simulink model "basis3"  (Simulink 6.6)
settings: Solver=ode45  StartTime=0.0  StopTime=inf  RelTol=1e-3
libraries: simulink x57, dspstat3 x3
settings Model: Creator=Paul.Dourbal  LastModifiedBy=Paul.Dourbal

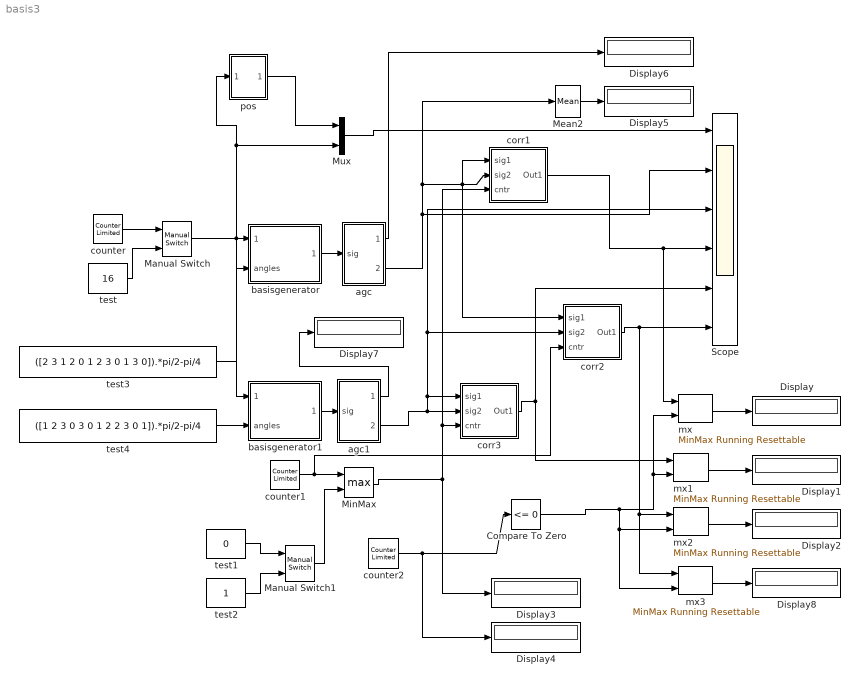
== system basis3 ==
  Compare To Zero : simulink/Logic and Bit Operations/Compare To Zero  SystemSampleTime=-1  relop=<=  LogicOutDataTypeMode=uint8  ZeroCross=off
  Display{,1..8} (9 alike) : Display
  Manual Switch : simulink/Signal Routing/Manual Switch  SystemSampleTime=-1  sw=1  action=0  varsize=off
  Manual Switch1 : simulink/Signal Routing/Manual Switch  SystemSampleTime=-1  sw=0  action=0  varsize=off
  Mean2 : dspstat3/Mean  DialogController=dspDDGCreate  DialogControllerArgs=DataTag0  run=on  reset_popup=None  roundingMode=Floor  overflowMode=on
  MinMax : MinMax  Function=max  Inputs=2  SampleTime=1
  Mux : Mux  Inputs=2
  Scope : Scope  NumInputPorts=6
      settings: TimeRange=102200  YMin=0~-1.25~-1.25~-0.1~-1~-1  YMax=70~1.25~1~1~1~2
  agc : Subsystem
  agc1 : Subsystem
  basisgenerator : Subsystem
  basisgenerator1 : Subsystem
  corr1 : Subsystem
  corr2 : Subsystem
  corr3 : Subsystem
  counter : simulink/Sources/Counter Limited  SystemSampleTime=-1  uplimit=2^(3+3)-1  tsamp=1
  counter1 : simulink/Sources/Counter Limited  SystemSampleTime=-1  uplimit=2^(3+3)-1  tsamp=256
  counter2 : simulink/Sources/Counter Limited  SystemSampleTime=-1  uplimit=2^(3+3)-1  tsamp=1024
  mx : simulink/Math Operations/MinMax Running Resettable  SystemSampleTime=-1  Function=max  vinit=0.0
  mx1 : simulink/Math Operations/MinMax Running Resettable  SystemSampleTime=-1  Function=max  vinit=0.0
  mx2 : simulink/Math Operations/MinMax Running Resettable  SystemSampleTime=-1  Function=max  vinit=0.0
  mx3 : simulink/Math Operations/MinMax Running Resettable  SystemSampleTime=-1  Function=min  vinit=0.0
  pos : Subsystem
  test : Constant  Value=16  OutDataTypeMode=uint8
  test1 : Constant  Value=0  OutDataTypeMode=uint8
  test2 : Constant  OutDataTypeMode=uint8
  test3 : Constant  Value=([2 3 1 2 0 1 2 3 0 1 3 0]).*pi/2-pi/4  OutDataTypeMode=double
  test4 : Constant  Value=([1 2 3 0 3 0 1 2 2 3 0 1]).*pi/2-pi/4  OutDataTypeMode=double
  wires:
  test/1 -> Manual Switch/2
  counter/1 -> Manual Switch/1
  Manual Switch/1 -> basisgenerator/1(counter), basisgenerator1/1(counter), pos/1(In1), Mux/2
  pos/1(Out1) -> Mux/1
  Mux/1 -> Scope/1
  corr1/1(Out1) -> Scope/4, mx/1
  corr3/1(Out1) -> Scope/5, mx1/1
  corr2/1(Out1) -> Scope/6, mx2/1, mx3/1
  counter1/1 -> MinMax/1, corr2/3(cntr)
  mx/1 -> Display/1
  mx1/1 -> Display1/1
  mx2/1 -> Display2/1
  Compare To Zero/1 -> mx/2, mx1/2, mx2/2, mx3/2
  counter2/1 -> Compare To Zero/1, Display4/1
  agc/2(out) -> Scope/2, corr1/2(sig2), corr1/1(sig1), corr2/1(sig1), Mean2/1
  agc1/2(out) -> Scope/3, corr2/2(sig2), corr3/1(sig1), corr3/2(sig2)
  Mean2/1 -> Display5/1
  agc/1(mean) -> Display6/1
  basisgenerator/1(samples) -> agc/1(sig)
  basisgenerator1/1(samples) -> agc1/1(sig)
  agc1/1(mean) -> Display7/1
  MinMax/1 -> corr1/3(cntr), corr3/3(cntr), Display3/1
  Manual Switch1/1 -> MinMax/2
  test1/1 -> Manual Switch1/1
  test2/1 -> Manual Switch1/2
  test4/1 -> basisgenerator1/2(angles)
  test3/1 -> basisgenerator/2(angles)
  mx3/1 -> Display8/1

== system basis3/agc ==
  sig : Inport
  Mean : dspstat3/Mean  DialogController=dspDDGCreate  DialogControllerArgs=DataTag1  run=on  reset_popup=None  roundingMode=Nearest  overflowMode=on
  Subtract : Sum  Inputs=+-  OutScaling=2^-10  SampleTime=1
  mean : Outport
  out : Outport  Port=2
  wires:
  sig/1 -> Subtract/1, Mean/1
  Mean/1 -> Subtract/2, mean/1
  Subtract/1 -> out/1

== system basis3/agc1 ==
  sig : Inport
  Mean : dspstat3/Mean  DialogController=dspDDGCreate  DialogControllerArgs=DataTag2  run=on  reset_popup=None  roundingMode=Nearest  overflowMode=on
  Subtract : Sum  Inputs=+-  OutScaling=2^-10  SampleTime=1
  mean : Outport
  out : Outport  Port=2
  wires:
  sig/1 -> Subtract/1, Mean/1
  Mean/1 -> Subtract/2, mean/1
  Subtract/1 -> out/1

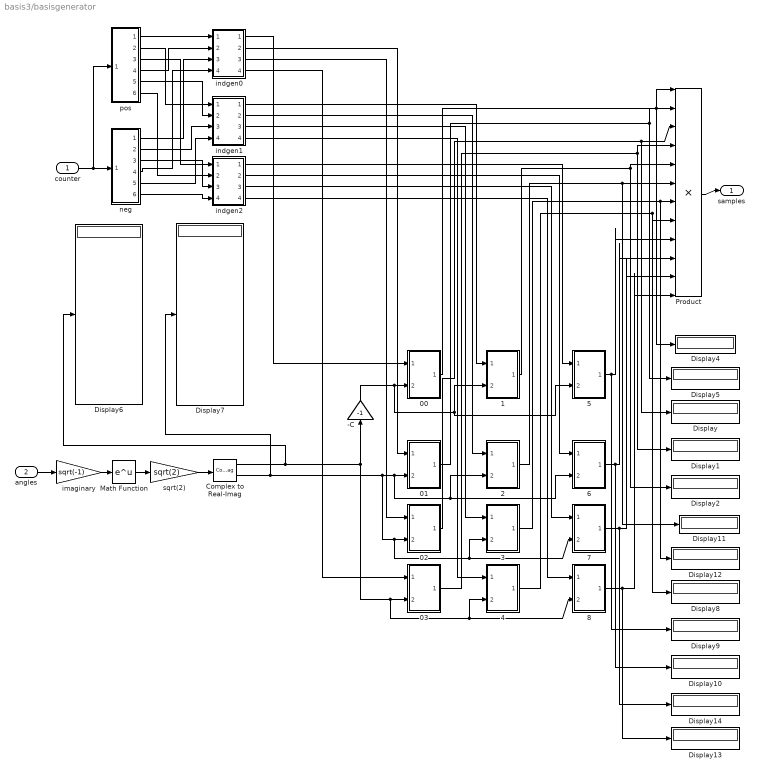
== system basis3/basisgenerator ==
  counter : Inport
  angles : Inport  Port=2
  -C : Gain  Orientation=up  Gain=-1
  00 : Subsystem
  01 : Subsystem
  02 : Subsystem
  03 : Subsystem
  1 : Subsystem
  2 : Subsystem
  3 : Subsystem
  4 : Subsystem
  5 : Subsystem
  6 : Subsystem
  7 : Subsystem
  8 : Subsystem
  Complex to Real-Imag : ComplexToRealImag
  Display{,1..2,4..14} (14 alike) : Display
  Math Function : Math  OutputSignalType=complex  SaturateOnIntegerOverflow=on
  Product : Product  Inputs=12  RndMeth=Zero
  imaginary : Gain  Gain=sqrt(-1)
  indgen0 : Subsystem
  indgen1 : Subsystem
  indgen2 : Subsystem
  neg : Subsystem
  pos : Subsystem
  sqrt(2) : Gain  Gain=sqrt(2)
  samples : Outport
  wires:
  8/1(Out1) -> Product/12, Display13/1
  7/1(Out1) -> Product/11, Display14/1
  6/1(Out1) -> Product/10, Display10/1
  5/1(Out1) -> Product/9, Display9/1
  4/1(Out1) -> Product/8, Display8/1
  3/1(Out1) -> Product/7, Display12/1
  2/1(Out1) -> Product/6, Display11/1
  1/1(Out1) -> Product/5, Display2/1
  03/1(Out1) -> Product/4, Display1/1
  02/1(Out1) -> Product/3, Display/1
  01/1(Out1) -> Product/2, Display5/1
  00/1(Out1) -> Product/1, Display4/1
  indgen2/4(Out4) -> 8/1(In1)
  indgen2/3(Out3) -> 7/1(In1)
  indgen2/2(Out2) -> 6/1(In1)
  indgen2/1(Out1) -> 5/1(In1)
  indgen1/4(Out4) -> 4/1(In1)
  indgen1/3(Out3) -> 3/1(In1)
  indgen1/2(Out2) -> 2/1(In1)
  indgen1/1(Out1) -> 1/1(In1)
  indgen0/4(Out4) -> 03/1(In1)
  indgen0/3(Out3) -> 02/1(In1)
  indgen0/2(Out2) -> 01/1(In1)
  indgen0/1(Out1) -> 00/1(In1)
  -C/1 -> 00/2(In2), 1/2(In2), 5/2(In2)
  neg/6(Out6) -> indgen2/4(In4)
  neg/3(Out3) -> indgen2/3(In3)
  pos/6(Out6) -> indgen2/2(In2)
  pos/3(Out3) -> indgen2/1(In1)
  neg/5(Out5) -> indgen1/4(In4)
  neg/2(Out2) -> indgen1/3(In3)
  pos/5(Out5) -> indgen1/2(In2)
  pos/2(Out2) -> indgen1/1(In1)
  neg/4(Out4) -> indgen0/4(In4)
  neg/1(Out1) -> indgen0/3(In3)
  pos/4(Out4) -> indgen0/2(In2)
  pos/1(Out1) -> indgen0/1(In1)
  Complex to Real-Imag/2 -> 01/2(In2), 2/2(In2), 6/2(In2), 02/2(In2), 3/2(In2), 7/2(In2), Display7/1
  Complex to Real-Imag/1 -> -C/1, 03/2(In2), 4/2(In2), 8/2(In2), Display6/1
  sqrt(2)/1 -> Complex to Real-Imag/1
  Math Function/1 -> sqrt(2)/1
  imaginary/1 -> Math Function/1
  counter/1 -> neg/1(In1), pos/1(In1)
  Product/1 -> samples/1
  angles/1 -> imaginary/1

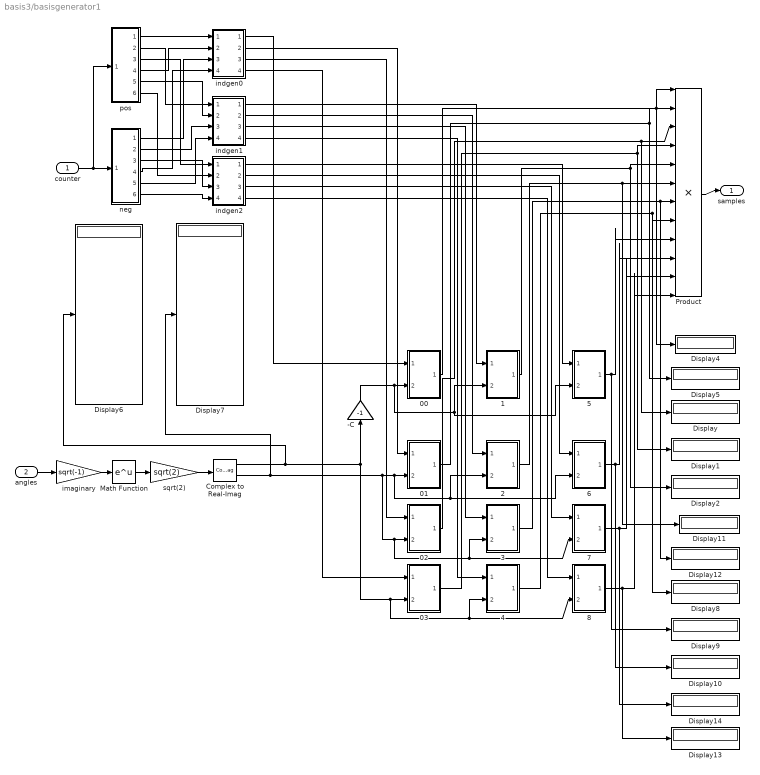
== system basis3/basisgenerator1 ==
  counter : Inport
  angles : Inport  Port=2
  -C : Gain  Orientation=up  Gain=-1
  00 : Subsystem
  01 : Subsystem
  02 : Subsystem
  03 : Subsystem
  1 : Subsystem
  2 : Subsystem
  3 : Subsystem
  4 : Subsystem
  5 : Subsystem
  6 : Subsystem
  7 : Subsystem
  8 : Subsystem
  Complex to Real-Imag : ComplexToRealImag
  Display{,1..2,4..14} (14 alike) : Display
  Math Function : Math  OutputSignalType=complex  SaturateOnIntegerOverflow=on
  Product : Product  Inputs=12  RndMeth=Zero
  imaginary : Gain  Gain=sqrt(-1)
  indgen0 : Subsystem
  indgen1 : Subsystem
  indgen2 : Subsystem
  neg : Subsystem
  pos : Subsystem
  sqrt(2) : Gain  Gain=sqrt(2)
  samples : Outport
  wires:
  8/1(Out1) -> Product/12, Display13/1
  7/1(Out1) -> Product/11, Display14/1
  6/1(Out1) -> Product/10, Display10/1
  5/1(Out1) -> Product/9, Display9/1
  4/1(Out1) -> Product/8, Display8/1
  3/1(Out1) -> Product/7, Display12/1
  2/1(Out1) -> Product/6, Display11/1
  1/1(Out1) -> Product/5, Display2/1
  03/1(Out1) -> Product/4, Display1/1
  02/1(Out1) -> Product/3, Display/1
  01/1(Out1) -> Product/2, Display5/1
  00/1(Out1) -> Product/1, Display4/1
  indgen2/4(Out4) -> 8/1(In1)
  indgen2/3(Out3) -> 7/1(In1)
  indgen2/2(Out2) -> 6/1(In1)
  indgen2/1(Out1) -> 5/1(In1)
  indgen1/4(Out4) -> 4/1(In1)
  indgen1/3(Out3) -> 3/1(In1)
  indgen1/2(Out2) -> 2/1(In1)
  indgen1/1(Out1) -> 1/1(In1)
  indgen0/4(Out4) -> 03/1(In1)
  indgen0/3(Out3) -> 02/1(In1)
  indgen0/2(Out2) -> 01/1(In1)
  indgen0/1(Out1) -> 00/1(In1)
  -C/1 -> 00/2(In2), 1/2(In2), 5/2(In2)
  neg/6(Out6) -> indgen2/4(In4)
  neg/3(Out3) -> indgen2/3(In3)
  pos/6(Out6) -> indgen2/2(In2)
  pos/3(Out3) -> indgen2/1(In1)
  neg/5(Out5) -> indgen1/4(In4)
  neg/2(Out2) -> indgen1/3(In3)
  pos/5(Out5) -> indgen1/2(In2)
  pos/2(Out2) -> indgen1/1(In1)
  neg/4(Out4) -> indgen0/4(In4)
  neg/1(Out1) -> indgen0/3(In3)
  pos/4(Out4) -> indgen0/2(In2)
  pos/1(Out1) -> indgen0/1(In1)
  Complex to Real-Imag/2 -> 01/2(In2), 2/2(In2), 6/2(In2), 02/2(In2), 3/2(In2), 7/2(In2), Display7/1
  Complex to Real-Imag/1 -> -C/1, 03/2(In2), 4/2(In2), 8/2(In2), Display6/1
  sqrt(2)/1 -> Complex to Real-Imag/1
  Math Function/1 -> sqrt(2)/1
  imaginary/1 -> Math Function/1
  counter/1 -> neg/1(In1), pos/1(In1)
  Product/1 -> samples/1
  angles/1 -> imaginary/1

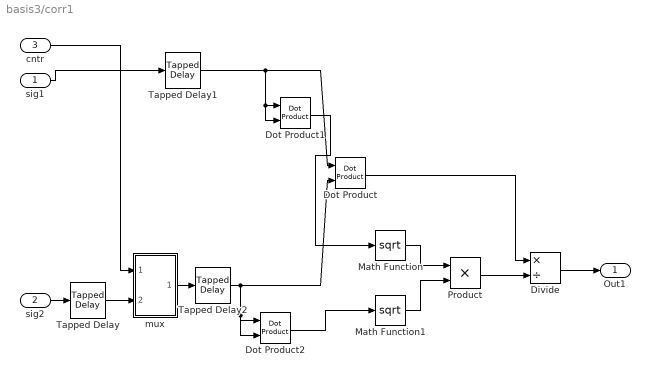
== system basis3/corr1 ==
  sig1 : Inport
  sig2 : Inport  Port=2
  cntr : Inport  Port=3
  Divide : Product  Inputs=*/  OutScaling=2^-10
  Dot Product : simulink/Math Operations/Dot Product  InputSameDT=on  OutDataType=sfix(16)  OutScaling=2^-10  DoSatur=off
  Dot Product1 : simulink/Math Operations/Dot Product  InputSameDT=on  OutDataType=sfix(16)  OutScaling=2^-10  DoSatur=off
  Dot Product2 : simulink/Math Operations/Dot Product  InputSameDT=on  OutDataType=sfix(16)  OutScaling=2^-10  DoSatur=off
  Math Function : Math  Operator=sqrt  SaturateOnIntegerOverflow=on
  Math Function1 : Math  Operator=sqrt  SaturateOnIntegerOverflow=on
  Product : Product  RndMeth=Zero
  Tapped Delay : simulink/Discrete/Tapped Delay  vinit=0.0  samptime=1  NumDelays=64  DelayOrder=Oldest  includeCurrent=off
  Tapped Delay1 : simulink/Discrete/Tapped Delay  vinit=0.0  samptime=1  NumDelays=64  DelayOrder=Oldest  includeCurrent=off
  Tapped Delay2 : simulink/Discrete/Tapped Delay  vinit=0.0  samptime=1  NumDelays=64  DelayOrder=Oldest  includeCurrent=off
  mux : Subsystem
  Out1 : Outport
  wires:
  Divide/1 -> Out1/1
  sig1/1 -> Tapped Delay1/1
  sig2/1 -> Tapped Delay/1
  Tapped Delay/1 -> mux/2(In2)
  cntr/1 -> mux/1(In1)
  mux/1(Out1) -> Tapped Delay2/1
  Tapped Delay1/1 -> Dot Product/1, Dot Product1/1, Dot Product1/2
  Tapped Delay2/1 -> Dot Product/2, Dot Product2/2, Dot Product2/1
  Math Function/1 -> Product/1
  Math Function1/1 -> Product/2
  Product/1 -> Divide/2
  Dot Product1/1 -> Math Function/1
  Dot Product2/1 -> Math Function1/1
  Dot Product/1 -> Divide/1

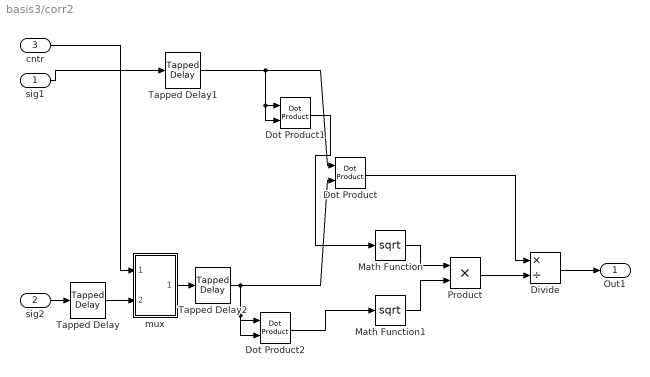
== system basis3/corr2 ==
  sig1 : Inport
  sig2 : Inport  Port=2
  cntr : Inport  Port=3
  Divide : Product  Inputs=*/  OutScaling=2^-10
  Dot Product : simulink/Math Operations/Dot Product  InputSameDT=on  OutDataType=sfix(16)  OutScaling=2^-10  DoSatur=off
  Dot Product1 : simulink/Math Operations/Dot Product  InputSameDT=on  OutDataType=sfix(16)  OutScaling=2^-10  DoSatur=off
  Dot Product2 : simulink/Math Operations/Dot Product  InputSameDT=on  OutDataType=sfix(16)  OutScaling=2^-10  DoSatur=off
  Math Function : Math  Operator=sqrt  SaturateOnIntegerOverflow=on
  Math Function1 : Math  Operator=sqrt  SaturateOnIntegerOverflow=on
  Product : Product  RndMeth=Zero
  Tapped Delay : simulink/Discrete/Tapped Delay  vinit=0.0  samptime=1  NumDelays=64  DelayOrder=Oldest  includeCurrent=off
  Tapped Delay1 : simulink/Discrete/Tapped Delay  vinit=0.0  samptime=1  NumDelays=64  DelayOrder=Oldest  includeCurrent=off
  Tapped Delay2 : simulink/Discrete/Tapped Delay  vinit=0.0  samptime=1  NumDelays=64  DelayOrder=Oldest  includeCurrent=off
  mux : Subsystem
  Out1 : Outport
  wires:
  Divide/1 -> Out1/1
  sig1/1 -> Tapped Delay1/1
  sig2/1 -> Tapped Delay/1
  Tapped Delay/1 -> mux/2(In2)
  cntr/1 -> mux/1(In1)
  mux/1(Out1) -> Tapped Delay2/1
  Tapped Delay1/1 -> Dot Product/1, Dot Product1/1, Dot Product1/2
  Tapped Delay2/1 -> Dot Product/2, Dot Product2/2, Dot Product2/1
  Math Function/1 -> Product/1
  Math Function1/1 -> Product/2
  Product/1 -> Divide/2
  Dot Product1/1 -> Math Function/1
  Dot Product2/1 -> Math Function1/1
  Dot Product/1 -> Divide/1

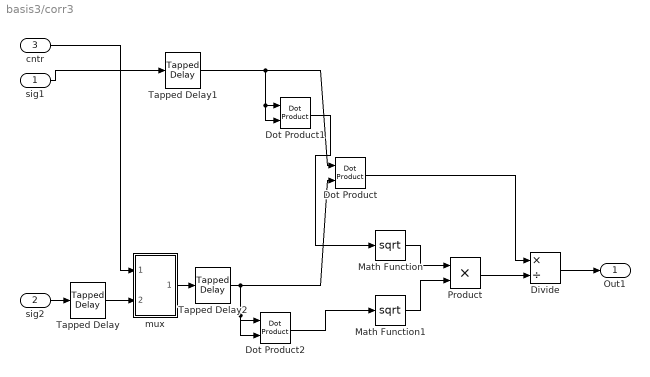
== system basis3/corr3 ==
  sig1 : Inport
  sig2 : Inport  Port=2
  cntr : Inport  Port=3
  Divide : Product  Inputs=*/  OutScaling=2^-10
  Dot Product : simulink/Math Operations/Dot Product  InputSameDT=on  OutDataType=sfix(16)  OutScaling=2^-10  DoSatur=off
  Dot Product1 : simulink/Math Operations/Dot Product  InputSameDT=on  OutDataType=sfix(16)  OutScaling=2^-10  DoSatur=off
  Dot Product2 : simulink/Math Operations/Dot Product  InputSameDT=on  OutDataType=sfix(16)  OutScaling=2^-10  DoSatur=off
  Math Function : Math  Operator=sqrt  SaturateOnIntegerOverflow=on
  Math Function1 : Math  Operator=sqrt  SaturateOnIntegerOverflow=on
  Product : Product  RndMeth=Zero
  Tapped Delay : simulink/Discrete/Tapped Delay  vinit=0.0  samptime=1  NumDelays=64  DelayOrder=Oldest  includeCurrent=off
  Tapped Delay1 : simulink/Discrete/Tapped Delay  vinit=0.0  samptime=1  NumDelays=64  DelayOrder=Oldest  includeCurrent=off
  Tapped Delay2 : simulink/Discrete/Tapped Delay  vinit=0.0  samptime=1  NumDelays=64  DelayOrder=Oldest  includeCurrent=off
  mux : Subsystem
  Out1 : Outport
  wires:
  Divide/1 -> Out1/1
  sig1/1 -> Tapped Delay1/1
  sig2/1 -> Tapped Delay/1
  Tapped Delay/1 -> mux/2(In2)
  cntr/1 -> mux/1(In1)
  mux/1(Out1) -> Tapped Delay2/1
  Tapped Delay1/1 -> Dot Product/1, Dot Product1/1, Dot Product1/2
  Tapped Delay2/1 -> Dot Product/2, Dot Product2/2, Dot Product2/1
  Math Function/1 -> Product/1
  Math Function1/1 -> Product/2
  Product/1 -> Divide/2
  Dot Product1/1 -> Math Function/1
  Dot Product2/1 -> Math Function1/1
  Dot Product/1 -> Divide/1

== system basis3/pos ==
  In1 : Inport  Orientation=up
  Extract Bits3 : simulink/Logic and Bit Operations/Extract Bits  SystemSampleTime=-1  bitsToExtract=Range of bits  numBits=8  bitIdxRange=[2 2]  outScalingMode=Treat bit field as an integer
  Extract Bits4 : simulink/Logic and Bit Operations/Extract Bits  SystemSampleTime=-1  bitsToExtract=Range of bits  numBits=8  bitIdxRange=[1 1]  outScalingMode=Treat bit field as an integer
  Extract Bits5 : simulink/Logic and Bit Operations/Extract Bits  SystemSampleTime=-1  bitsToExtract=Range of bits  numBits=8  bitIdxRange=[0 0]  outScalingMode=Treat bit field as an integer
  ws : Subsystem
  Out1 : Outport
  wires:
  Extract Bits5/1 -> ws/1(in0)
  In1/1 -> Extract Bits3/1, Extract Bits5/1, Extract Bits4/1
  Extract Bits4/1 -> ws/2(in1)
  Extract Bits3/1 -> ws/3(in2)
  ws/1(Out1) -> Out1/1

== system basis3/basisgenerator/00 ==
  In1 : Inport
  In2 : Inport  Port=2
  C : MultiPortSwitch  Inputs=12  zeroidx=on
  Demux3 : Demux  Outputs=12
  Out1 : Outport
  wires:
  Demux3/1 -> C/2
  Demux3/2 -> C/3
  Demux3/3 -> C/4
  Demux3/4 -> C/5
  Demux3/5 -> C/6
  Demux3/6 -> C/7
  Demux3/7 -> C/8
  Demux3/8 -> C/9
  Demux3/9 -> C/10
  Demux3/10 -> C/11
  Demux3/11 -> C/12
  Demux3/12 -> C/13
  In1/1 -> C/1
  C/1 -> Out1/1
  In2/1 -> Demux3/1

== system basis3/basisgenerator/01 ==
  In1 : Inport
  In2 : Inport  Port=2
  C : MultiPortSwitch  Inputs=12  zeroidx=on
  Demux3 : Demux  Outputs=12
  Out1 : Outport
  wires:
  Demux3/1 -> C/2
  Demux3/2 -> C/3
  Demux3/3 -> C/4
  Demux3/4 -> C/5
  Demux3/5 -> C/6
  Demux3/6 -> C/7
  Demux3/7 -> C/8
  Demux3/8 -> C/9
  Demux3/9 -> C/10
  Demux3/10 -> C/11
  Demux3/11 -> C/12
  Demux3/12 -> C/13
  In1/1 -> C/1
  C/1 -> Out1/1
  In2/1 -> Demux3/1

== system basis3/basisgenerator/02 ==
  In1 : Inport
  In2 : Inport  Port=2
  C : MultiPortSwitch  Inputs=12  zeroidx=on
  Demux3 : Demux  Outputs=12
  Out1 : Outport
  wires:
  Demux3/1 -> C/2
  Demux3/2 -> C/3
  Demux3/3 -> C/4
  Demux3/4 -> C/5
  Demux3/5 -> C/6
  Demux3/6 -> C/7
  Demux3/7 -> C/8
  Demux3/8 -> C/9
  Demux3/9 -> C/10
  Demux3/10 -> C/11
  Demux3/11 -> C/12
  Demux3/12 -> C/13
  In1/1 -> C/1
  C/1 -> Out1/1
  In2/1 -> Demux3/1

== system basis3/basisgenerator/03 ==
  In1 : Inport
  In2 : Inport  Port=2
  C : MultiPortSwitch  Inputs=12  zeroidx=on
  Demux3 : Demux  Outputs=12
  Out1 : Outport
  wires:
  Demux3/1 -> C/2
  Demux3/2 -> C/3
  Demux3/3 -> C/4
  Demux3/4 -> C/5
  Demux3/5 -> C/6
  Demux3/6 -> C/7
  Demux3/7 -> C/8
  Demux3/8 -> C/9
  Demux3/9 -> C/10
  Demux3/10 -> C/11
  Demux3/11 -> C/12
  Demux3/12 -> C/13
  In1/1 -> C/1
  C/1 -> Out1/1
  In2/1 -> Demux3/1

== system basis3/basisgenerator/1 ==
  In1 : Inport
  In2 : Inport  Port=2
  C : MultiPortSwitch  Inputs=12  zeroidx=on
  Demux3 : Demux  Outputs=12
  Out1 : Outport
  wires:
  Demux3/1 -> C/2
  Demux3/2 -> C/3
  Demux3/3 -> C/4
  Demux3/4 -> C/5
  Demux3/5 -> C/6
  Demux3/6 -> C/7
  Demux3/7 -> C/8
  Demux3/8 -> C/9
  Demux3/9 -> C/10
  Demux3/10 -> C/11
  Demux3/11 -> C/12
  Demux3/12 -> C/13
  In1/1 -> C/1
  C/1 -> Out1/1
  In2/1 -> Demux3/1

== system basis3/basisgenerator/2 ==
  In1 : Inport
  In2 : Inport  Port=2
  C : MultiPortSwitch  Inputs=12  zeroidx=on
  Demux3 : Demux  Outputs=12
  Out1 : Outport
  wires:
  Demux3/1 -> C/2
  Demux3/2 -> C/3
  Demux3/3 -> C/4
  Demux3/4 -> C/5
  Demux3/5 -> C/6
  Demux3/6 -> C/7
  Demux3/7 -> C/8
  Demux3/8 -> C/9
  Demux3/9 -> C/10
  Demux3/10 -> C/11
  Demux3/11 -> C/12
  Demux3/12 -> C/13
  In1/1 -> C/1
  C/1 -> Out1/1
  In2/1 -> Demux3/1

== system basis3/basisgenerator/3 ==
  In1 : Inport
  In2 : Inport  Port=2
  C : MultiPortSwitch  Inputs=12  zeroidx=on
  Demux3 : Demux  Outputs=12
  Out1 : Outport
  wires:
  Demux3/1 -> C/2
  Demux3/2 -> C/3
  Demux3/3 -> C/4
  Demux3/4 -> C/5
  Demux3/5 -> C/6
  Demux3/6 -> C/7
  Demux3/7 -> C/8
  Demux3/8 -> C/9
  Demux3/9 -> C/10
  Demux3/10 -> C/11
  Demux3/11 -> C/12
  Demux3/12 -> C/13
  In1/1 -> C/1
  C/1 -> Out1/1
  In2/1 -> Demux3/1

== system basis3/basisgenerator/4 ==
  In1 : Inport
  In2 : Inport  Port=2
  C : MultiPortSwitch  Inputs=12  zeroidx=on
  Demux3 : Demux  Outputs=12
  Out1 : Outport
  wires:
  Demux3/1 -> C/2
  Demux3/2 -> C/3
  Demux3/3 -> C/4
  Demux3/4 -> C/5
  Demux3/5 -> C/6
  Demux3/6 -> C/7
  Demux3/7 -> C/8
  Demux3/8 -> C/9
  Demux3/9 -> C/10
  Demux3/10 -> C/11
  Demux3/11 -> C/12
  Demux3/12 -> C/13
  In1/1 -> C/1
  C/1 -> Out1/1
  In2/1 -> Demux3/1

== system basis3/basisgenerator/5 ==
  In1 : Inport
  In2 : Inport  Port=2
  C : MultiPortSwitch  Inputs=12  zeroidx=on
  Demux3 : Demux  Outputs=12
  Out1 : Outport
  wires:
  Demux3/1 -> C/2
  Demux3/2 -> C/3
  Demux3/3 -> C/4
  Demux3/4 -> C/5
  Demux3/5 -> C/6
  Demux3/6 -> C/7
  Demux3/7 -> C/8
  Demux3/8 -> C/9
  Demux3/9 -> C/10
  Demux3/10 -> C/11
  Demux3/11 -> C/12
  Demux3/12 -> C/13
  In1/1 -> C/1
  C/1 -> Out1/1
  In2/1 -> Demux3/1

== system basis3/basisgenerator/6 ==
  In1 : Inport
  In2 : Inport  Port=2
  C : MultiPortSwitch  Inputs=12  zeroidx=on
  Demux3 : Demux  Outputs=12
  Out1 : Outport
  wires:
  Demux3/1 -> C/2
  Demux3/2 -> C/3
  Demux3/3 -> C/4
  Demux3/4 -> C/5
  Demux3/5 -> C/6
  Demux3/6 -> C/7
  Demux3/7 -> C/8
  Demux3/8 -> C/9
  Demux3/9 -> C/10
  Demux3/10 -> C/11
  Demux3/11 -> C/12
  Demux3/12 -> C/13
  In1/1 -> C/1
  C/1 -> Out1/1
  In2/1 -> Demux3/1

== system basis3/basisgenerator/7 ==
  In1 : Inport
  In2 : Inport  Port=2
  C : MultiPortSwitch  Inputs=12  zeroidx=on
  Demux3 : Demux  Outputs=12
  Out1 : Outport
  wires:
  Demux3/1 -> C/2
  Demux3/2 -> C/3
  Demux3/3 -> C/4
  Demux3/4 -> C/5
  Demux3/5 -> C/6
  Demux3/6 -> C/7
  Demux3/7 -> C/8
  Demux3/8 -> C/9
  Demux3/9 -> C/10
  Demux3/10 -> C/11
  Demux3/11 -> C/12
  Demux3/12 -> C/13
  In1/1 -> C/1
  C/1 -> Out1/1
  In2/1 -> Demux3/1

== system basis3/basisgenerator/8 ==
  In1 : Inport
  In2 : Inport  Port=2
  C : MultiPortSwitch  Inputs=12  zeroidx=on
  Demux3 : Demux  Outputs=12
  Out1 : Outport
  wires:
  Demux3/1 -> C/2
  Demux3/2 -> C/3
  Demux3/3 -> C/4
  Demux3/4 -> C/5
  Demux3/5 -> C/6
  Demux3/6 -> C/7
  Demux3/7 -> C/8
  Demux3/8 -> C/9
  Demux3/9 -> C/10
  Demux3/10 -> C/11
  Demux3/11 -> C/12
  Demux3/12 -> C/13
  In1/1 -> C/1
  C/1 -> Out1/1
  In2/1 -> Demux3/1

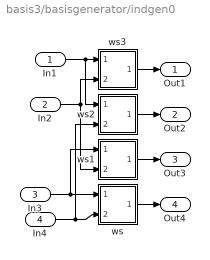
== system basis3/basisgenerator/indgen0 ==
  In1 : Inport
  In2 : Inport  Port=2
  In3 : Inport  Port=3
  In4 : Inport  Port=4
  ws : Subsystem
  ws1 : Subsystem
  ws2 : Subsystem
  ws3 : Subsystem
  Out1 : Outport
  Out2 : Outport  Port=2
  Out3 : Outport  Port=3
  Out4 : Outport  Port=4
  wires:
  In3/1 -> ws1/1(In1), ws/1(In1)
  In4/1 -> ws2/2(In2), ws/2(In2)
  In2/1 -> ws3/2(In2), ws1/2(In2)
  In1/1 -> ws3/1(In1), ws2/1(In1)
  ws3/1(Out1) -> Out1/1
  ws2/1(Out1) -> Out2/1
  ws1/1(Out1) -> Out3/1
  ws/1(Out1) -> Out4/1

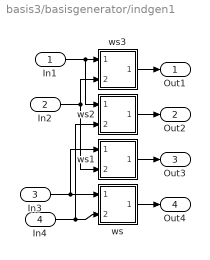
== system basis3/basisgenerator/indgen1 ==
  In1 : Inport
  In2 : Inport  Port=2
  In3 : Inport  Port=3
  In4 : Inport  Port=4
  ws : Subsystem
  ws1 : Subsystem
  ws2 : Subsystem
  ws3 : Subsystem
  Out1 : Outport
  Out2 : Outport  Port=2
  Out3 : Outport  Port=3
  Out4 : Outport  Port=4
  wires:
  In3/1 -> ws1/1(In1), ws/1(In1)
  In4/1 -> ws2/2(In2), ws/2(In2)
  In2/1 -> ws3/2(In2), ws1/2(In2)
  In1/1 -> ws3/1(In1), ws2/1(In1)
  ws3/1(Out1) -> Out1/1
  ws2/1(Out1) -> Out2/1
  ws1/1(Out1) -> Out3/1
  ws/1(Out1) -> Out4/1

== system basis3/basisgenerator/indgen2 ==
  In1 : Inport
  In2 : Inport  Port=2
  In3 : Inport  Port=3
  In4 : Inport  Port=4
  ws : Subsystem
  ws1 : Subsystem
  ws2 : Subsystem
  ws3 : Subsystem
  Out1 : Outport
  Out2 : Outport  Port=2
  Out3 : Outport  Port=3
  Out4 : Outport  Port=4
  wires:
  In3/1 -> ws1/1(In1), ws/1(In1)
  In4/1 -> ws2/2(In2), ws/2(In2)
  In2/1 -> ws3/2(In2), ws1/2(In2)
  In1/1 -> ws3/1(In1), ws2/1(In1)
  ws3/1(Out1) -> Out1/1
  ws2/1(Out1) -> Out2/1
  ws1/1(Out1) -> Out3/1
  ws/1(Out1) -> Out4/1

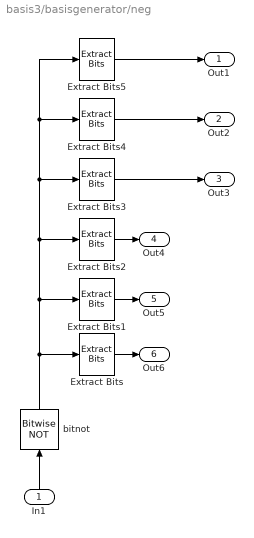
== system basis3/basisgenerator/neg ==
  In1 : Inport  Orientation=up
  Extract Bits : simulink/Logic and Bit Operations/Extract Bits  SystemSampleTime=-1  bitsToExtract=Range of bits  numBits=8  bitIdxRange=[5 5]  outScalingMode=Treat bit field as an integer
  Extract Bits1 : simulink/Logic and Bit Operations/Extract Bits  SystemSampleTime=-1  bitsToExtract=Range of bits  numBits=8  bitIdxRange=[4 4]  outScalingMode=Treat bit field as an integer
  Extract Bits2 : simulink/Logic and Bit Operations/Extract Bits  SystemSampleTime=-1  bitsToExtract=Range of bits  numBits=8  bitIdxRange=[3 3]  outScalingMode=Treat bit field as an integer
  Extract Bits3 : simulink/Logic and Bit Operations/Extract Bits  SystemSampleTime=-1  bitsToExtract=Range of bits  numBits=8  bitIdxRange=[2 2]  outScalingMode=Treat bit field as an integer
  Extract Bits4 : simulink/Logic and Bit Operations/Extract Bits  SystemSampleTime=-1  bitsToExtract=Range of bits  numBits=8  bitIdxRange=[1 1]  outScalingMode=Treat bit field as an integer
  Extract Bits5 : simulink/Logic and Bit Operations/Extract Bits  SystemSampleTime=-1  bitsToExtract=Range of bits  numBits=8  bitIdxRange=[0 0]  outScalingMode=Treat bit field as an integer
  bitnot : simulink/Logic and Bit Operations/Bitwise Operator  Orientation=up  logicop=NOT  UseBitMask=off  BitMask=bin2dec('11011001')  BitMaskRealWorld=Stored Integer
  Out1 : Outport
  Out2 : Outport  Port=2
  Out3 : Outport  Port=3
  Out4 : Outport  Port=4
  Out5 : Outport  Port=5
  Out6 : Outport  Port=6
  wires:
  Extract Bits5/1 -> Out1/1
  Extract Bits4/1 -> Out2/1
  Extract Bits3/1 -> Out3/1
  Extract Bits2/1 -> Out4/1
  In1/1 -> bitnot/1
  Extract Bits1/1 -> Out5/1
  Extract Bits/1 -> Out6/1
  bitnot/1 -> Extract Bits1/1, Extract Bits2/1, Extract Bits3/1, Extract Bits5/1, Extract Bits4/1, Extract Bits/1

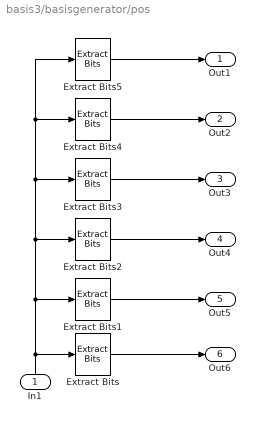
== system basis3/basisgenerator/pos ==
  In1 : Inport  Orientation=up
  Extract Bits : simulink/Logic and Bit Operations/Extract Bits  SystemSampleTime=-1  bitsToExtract=Range of bits  numBits=8  bitIdxRange=[5 5]  outScalingMode=Treat bit field as an integer
  Extract Bits1 : simulink/Logic and Bit Operations/Extract Bits  SystemSampleTime=-1  bitsToExtract=Range of bits  numBits=8  bitIdxRange=[4 4]  outScalingMode=Treat bit field as an integer
  Extract Bits2 : simulink/Logic and Bit Operations/Extract Bits  SystemSampleTime=-1  bitsToExtract=Range of bits  numBits=8  bitIdxRange=[3 3]  outScalingMode=Treat bit field as an integer
  Extract Bits3 : simulink/Logic and Bit Operations/Extract Bits  SystemSampleTime=-1  bitsToExtract=Range of bits  numBits=8  bitIdxRange=[2 2]  outScalingMode=Treat bit field as an integer
  Extract Bits4 : simulink/Logic and Bit Operations/Extract Bits  SystemSampleTime=-1  bitsToExtract=Range of bits  numBits=8  bitIdxRange=[1 1]  outScalingMode=Treat bit field as an integer
  Extract Bits5 : simulink/Logic and Bit Operations/Extract Bits  SystemSampleTime=-1  bitsToExtract=Range of bits  numBits=8  bitIdxRange=[0 0]  outScalingMode=Treat bit field as an integer
  Out1 : Outport
  Out2 : Outport  Port=2
  Out3 : Outport  Port=3
  Out4 : Outport  Port=4
  Out5 : Outport  Port=5
  Out6 : Outport  Port=6
  wires:
  Extract Bits5/1 -> Out1/1
  Extract Bits4/1 -> Out2/1
  Extract Bits3/1 -> Out3/1
  Extract Bits2/1 -> Out4/1
  In1/1 -> Extract Bits1/1, Extract Bits2/1, Extract Bits3/1, Extract Bits5/1, Extract Bits4/1, Extract Bits/1
  Extract Bits1/1 -> Out5/1
  Extract Bits/1 -> Out6/1

== system basis3/basisgenerator1/00 ==
  In1 : Inport
  In2 : Inport  Port=2
  C : MultiPortSwitch  Inputs=12  zeroidx=on
  Demux3 : Demux  Outputs=12
  Out1 : Outport
  wires:
  Demux3/1 -> C/2
  Demux3/2 -> C/3
  Demux3/3 -> C/4
  Demux3/4 -> C/5
  Demux3/5 -> C/6
  Demux3/6 -> C/7
  Demux3/7 -> C/8
  Demux3/8 -> C/9
  Demux3/9 -> C/10
  Demux3/10 -> C/11
  Demux3/11 -> C/12
  Demux3/12 -> C/13
  In1/1 -> C/1
  C/1 -> Out1/1
  In2/1 -> Demux3/1

== system basis3/basisgenerator1/01 ==
  In1 : Inport
  In2 : Inport  Port=2
  C : MultiPortSwitch  Inputs=12  zeroidx=on
  Demux3 : Demux  Outputs=12
  Out1 : Outport
  wires:
  Demux3/1 -> C/2
  Demux3/2 -> C/3
  Demux3/3 -> C/4
  Demux3/4 -> C/5
  Demux3/5 -> C/6
  Demux3/6 -> C/7
  Demux3/7 -> C/8
  Demux3/8 -> C/9
  Demux3/9 -> C/10
  Demux3/10 -> C/11
  Demux3/11 -> C/12
  Demux3/12 -> C/13
  In1/1 -> C/1
  C/1 -> Out1/1
  In2/1 -> Demux3/1

== system basis3/basisgenerator1/02 ==
  In1 : Inport
  In2 : Inport  Port=2
  C : MultiPortSwitch  Inputs=12  zeroidx=on
  Demux3 : Demux  Outputs=12
  Out1 : Outport
  wires:
  Demux3/1 -> C/2
  Demux3/2 -> C/3
  Demux3/3 -> C/4
  Demux3/4 -> C/5
  Demux3/5 -> C/6
  Demux3/6 -> C/7
  Demux3/7 -> C/8
  Demux3/8 -> C/9
  Demux3/9 -> C/10
  Demux3/10 -> C/11
  Demux3/11 -> C/12
  Demux3/12 -> C/13
  In1/1 -> C/1
  C/1 -> Out1/1
  In2/1 -> Demux3/1

== system basis3/basisgenerator1/03 ==
  In1 : Inport
  In2 : Inport  Port=2
  C : MultiPortSwitch  Inputs=12  zeroidx=on
  Demux3 : Demux  Outputs=12
  Out1 : Outport
  wires:
  Demux3/1 -> C/2
  Demux3/2 -> C/3
  Demux3/3 -> C/4
  Demux3/4 -> C/5
  Demux3/5 -> C/6
  Demux3/6 -> C/7
  Demux3/7 -> C/8
  Demux3/8 -> C/9
  Demux3/9 -> C/10
  Demux3/10 -> C/11
  Demux3/11 -> C/12
  Demux3/12 -> C/13
  In1/1 -> C/1
  C/1 -> Out1/1
  In2/1 -> Demux3/1

== system basis3/basisgenerator1/1 ==
  In1 : Inport
  In2 : Inport  Port=2
  C : MultiPortSwitch  Inputs=12  zeroidx=on
  Demux3 : Demux  Outputs=12
  Out1 : Outport
  wires:
  Demux3/1 -> C/2
  Demux3/2 -> C/3
  Demux3/3 -> C/4
  Demux3/4 -> C/5
  Demux3/5 -> C/6
  Demux3/6 -> C/7
  Demux3/7 -> C/8
  Demux3/8 -> C/9
  Demux3/9 -> C/10
  Demux3/10 -> C/11
  Demux3/11 -> C/12
  Demux3/12 -> C/13
  In1/1 -> C/1
  C/1 -> Out1/1
  In2/1 -> Demux3/1

== system basis3/basisgenerator1/2 ==
  In1 : Inport
  In2 : Inport  Port=2
  C : MultiPortSwitch  Inputs=12  zeroidx=on
  Demux3 : Demux  Outputs=12
  Out1 : Outport
  wires:
  Demux3/1 -> C/2
  Demux3/2 -> C/3
  Demux3/3 -> C/4
  Demux3/4 -> C/5
  Demux3/5 -> C/6
  Demux3/6 -> C/7
  Demux3/7 -> C/8
  Demux3/8 -> C/9
  Demux3/9 -> C/10
  Demux3/10 -> C/11
  Demux3/11 -> C/12
  Demux3/12 -> C/13
  In1/1 -> C/1
  C/1 -> Out1/1
  In2/1 -> Demux3/1

== system basis3/basisgenerator1/3 ==
  In1 : Inport
  In2 : Inport  Port=2
  C : MultiPortSwitch  Inputs=12  zeroidx=on
  Demux3 : Demux  Outputs=12
  Out1 : Outport
  wires:
  Demux3/1 -> C/2
  Demux3/2 -> C/3
  Demux3/3 -> C/4
  Demux3/4 -> C/5
  Demux3/5 -> C/6
  Demux3/6 -> C/7
  Demux3/7 -> C/8
  Demux3/8 -> C/9
  Demux3/9 -> C/10
  Demux3/10 -> C/11
  Demux3/11 -> C/12
  Demux3/12 -> C/13
  In1/1 -> C/1
  C/1 -> Out1/1
  In2/1 -> Demux3/1

== system basis3/basisgenerator1/4 ==
  In1 : Inport
  In2 : Inport  Port=2
  C : MultiPortSwitch  Inputs=12  zeroidx=on
  Demux3 : Demux  Outputs=12
  Out1 : Outport
  wires:
  Demux3/1 -> C/2
  Demux3/2 -> C/3
  Demux3/3 -> C/4
  Demux3/4 -> C/5
  Demux3/5 -> C/6
  Demux3/6 -> C/7
  Demux3/7 -> C/8
  Demux3/8 -> C/9
  Demux3/9 -> C/10
  Demux3/10 -> C/11
  Demux3/11 -> C/12
  Demux3/12 -> C/13
  In1/1 -> C/1
  C/1 -> Out1/1
  In2/1 -> Demux3/1

== system basis3/basisgenerator1/5 ==
  In1 : Inport
  In2 : Inport  Port=2
  C : MultiPortSwitch  Inputs=12  zeroidx=on
  Demux3 : Demux  Outputs=12
  Out1 : Outport
  wires:
  Demux3/1 -> C/2
  Demux3/2 -> C/3
  Demux3/3 -> C/4
  Demux3/4 -> C/5
  Demux3/5 -> C/6
  Demux3/6 -> C/7
  Demux3/7 -> C/8
  Demux3/8 -> C/9
  Demux3/9 -> C/10
  Demux3/10 -> C/11
  Demux3/11 -> C/12
  Demux3/12 -> C/13
  In1/1 -> C/1
  C/1 -> Out1/1
  In2/1 -> Demux3/1

== system basis3/basisgenerator1/6 ==
  In1 : Inport
  In2 : Inport  Port=2
  C : MultiPortSwitch  Inputs=12  zeroidx=on
  Demux3 : Demux  Outputs=12
  Out1 : Outport
  wires:
  Demux3/1 -> C/2
  Demux3/2 -> C/3
  Demux3/3 -> C/4
  Demux3/4 -> C/5
  Demux3/5 -> C/6
  Demux3/6 -> C/7
  Demux3/7 -> C/8
  Demux3/8 -> C/9
  Demux3/9 -> C/10
  Demux3/10 -> C/11
  Demux3/11 -> C/12
  Demux3/12 -> C/13
  In1/1 -> C/1
  C/1 -> Out1/1
  In2/1 -> Demux3/1

== system basis3/basisgenerator1/7 ==
  In1 : Inport
  In2 : Inport  Port=2
  C : MultiPortSwitch  Inputs=12  zeroidx=on
  Demux3 : Demux  Outputs=12
  Out1 : Outport
  wires:
  Demux3/1 -> C/2
  Demux3/2 -> C/3
  Demux3/3 -> C/4
  Demux3/4 -> C/5
  Demux3/5 -> C/6
  Demux3/6 -> C/7
  Demux3/7 -> C/8
  Demux3/8 -> C/9
  Demux3/9 -> C/10
  Demux3/10 -> C/11
  Demux3/11 -> C/12
  Demux3/12 -> C/13
  In1/1 -> C/1
  C/1 -> Out1/1
  In2/1 -> Demux3/1

== system basis3/basisgenerator1/8 ==
  In1 : Inport
  In2 : Inport  Port=2
  C : MultiPortSwitch  Inputs=12  zeroidx=on
  Demux3 : Demux  Outputs=12
  Out1 : Outport
  wires:
  Demux3/1 -> C/2
  Demux3/2 -> C/3
  Demux3/3 -> C/4
  Demux3/4 -> C/5
  Demux3/5 -> C/6
  Demux3/6 -> C/7
  Demux3/7 -> C/8
  Demux3/8 -> C/9
  Demux3/9 -> C/10
  Demux3/10 -> C/11
  Demux3/11 -> C/12
  Demux3/12 -> C/13
  In1/1 -> C/1
  C/1 -> Out1/1
  In2/1 -> Demux3/1

== system basis3/basisgenerator1/indgen0 ==
  In1 : Inport
  In2 : Inport  Port=2
  In3 : Inport  Port=3
  In4 : Inport  Port=4
  ws : Subsystem
  ws1 : Subsystem
  ws2 : Subsystem
  ws3 : Subsystem
  Out1 : Outport
  Out2 : Outport  Port=2
  Out3 : Outport  Port=3
  Out4 : Outport  Port=4
  wires:
  In3/1 -> ws1/1(In1), ws/1(In1)
  In4/1 -> ws2/2(In2), ws/2(In2)
  In2/1 -> ws3/2(In2), ws1/2(In2)
  In1/1 -> ws3/1(In1), ws2/1(In1)
  ws3/1(Out1) -> Out1/1
  ws2/1(Out1) -> Out2/1
  ws1/1(Out1) -> Out3/1
  ws/1(Out1) -> Out4/1

== system basis3/basisgenerator1/indgen1 ==
  In1 : Inport
  In2 : Inport  Port=2
  In3 : Inport  Port=3
  In4 : Inport  Port=4
  ws : Subsystem
  ws1 : Subsystem
  ws2 : Subsystem
  ws3 : Subsystem
  Out1 : Outport
  Out2 : Outport  Port=2
  Out3 : Outport  Port=3
  Out4 : Outport  Port=4
  wires:
  In3/1 -> ws1/1(In1), ws/1(In1)
  In4/1 -> ws2/2(In2), ws/2(In2)
  In2/1 -> ws3/2(In2), ws1/2(In2)
  In1/1 -> ws3/1(In1), ws2/1(In1)
  ws3/1(Out1) -> Out1/1
  ws2/1(Out1) -> Out2/1
  ws1/1(Out1) -> Out3/1
  ws/1(Out1) -> Out4/1

== system basis3/basisgenerator1/indgen2 ==
  In1 : Inport
  In2 : Inport  Port=2
  In3 : Inport  Port=3
  In4 : Inport  Port=4
  ws : Subsystem
  ws1 : Subsystem
  ws2 : Subsystem
  ws3 : Subsystem
  Out1 : Outport
  Out2 : Outport  Port=2
  Out3 : Outport  Port=3
  Out4 : Outport  Port=4
  wires:
  In3/1 -> ws1/1(In1), ws/1(In1)
  In4/1 -> ws2/2(In2), ws/2(In2)
  In2/1 -> ws3/2(In2), ws1/2(In2)
  In1/1 -> ws3/1(In1), ws2/1(In1)
  ws3/1(Out1) -> Out1/1
  ws2/1(Out1) -> Out2/1
  ws1/1(Out1) -> Out3/1
  ws/1(Out1) -> Out4/1

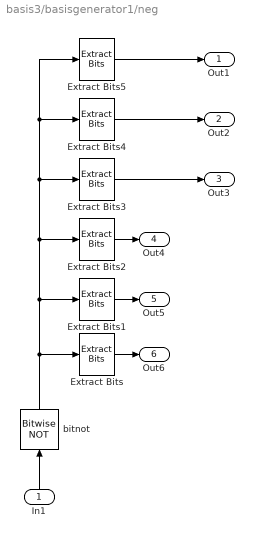
== system basis3/basisgenerator1/neg ==
  In1 : Inport  Orientation=up
  Extract Bits : simulink/Logic and Bit Operations/Extract Bits  SystemSampleTime=-1  bitsToExtract=Range of bits  numBits=8  bitIdxRange=[5 5]  outScalingMode=Treat bit field as an integer
  Extract Bits1 : simulink/Logic and Bit Operations/Extract Bits  SystemSampleTime=-1  bitsToExtract=Range of bits  numBits=8  bitIdxRange=[4 4]  outScalingMode=Treat bit field as an integer
  Extract Bits2 : simulink/Logic and Bit Operations/Extract Bits  SystemSampleTime=-1  bitsToExtract=Range of bits  numBits=8  bitIdxRange=[3 3]  outScalingMode=Treat bit field as an integer
  Extract Bits3 : simulink/Logic and Bit Operations/Extract Bits  SystemSampleTime=-1  bitsToExtract=Range of bits  numBits=8  bitIdxRange=[2 2]  outScalingMode=Treat bit field as an integer
  Extract Bits4 : simulink/Logic and Bit Operations/Extract Bits  SystemSampleTime=-1  bitsToExtract=Range of bits  numBits=8  bitIdxRange=[1 1]  outScalingMode=Treat bit field as an integer
  Extract Bits5 : simulink/Logic and Bit Operations/Extract Bits  SystemSampleTime=-1  bitsToExtract=Range of bits  numBits=8  bitIdxRange=[0 0]  outScalingMode=Treat bit field as an integer
  bitnot : simulink/Logic and Bit Operations/Bitwise Operator  Orientation=up  logicop=NOT  UseBitMask=off  BitMask=bin2dec('11011001')  BitMaskRealWorld=Stored Integer
  Out1 : Outport
  Out2 : Outport  Port=2
  Out3 : Outport  Port=3
  Out4 : Outport  Port=4
  Out5 : Outport  Port=5
  Out6 : Outport  Port=6
  wires:
  Extract Bits5/1 -> Out1/1
  Extract Bits4/1 -> Out2/1
  Extract Bits3/1 -> Out3/1
  Extract Bits2/1 -> Out4/1
  In1/1 -> bitnot/1
  Extract Bits1/1 -> Out5/1
  Extract Bits/1 -> Out6/1
  bitnot/1 -> Extract Bits1/1, Extract Bits2/1, Extract Bits3/1, Extract Bits5/1, Extract Bits4/1, Extract Bits/1

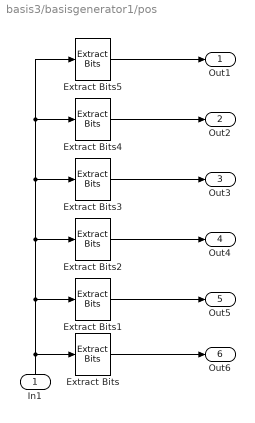
== system basis3/basisgenerator1/pos ==
  In1 : Inport  Orientation=up
  Extract Bits : simulink/Logic and Bit Operations/Extract Bits  SystemSampleTime=-1  bitsToExtract=Range of bits  numBits=8  bitIdxRange=[5 5]  outScalingMode=Treat bit field as an integer
  Extract Bits1 : simulink/Logic and Bit Operations/Extract Bits  SystemSampleTime=-1  bitsToExtract=Range of bits  numBits=8  bitIdxRange=[4 4]  outScalingMode=Treat bit field as an integer
  Extract Bits2 : simulink/Logic and Bit Operations/Extract Bits  SystemSampleTime=-1  bitsToExtract=Range of bits  numBits=8  bitIdxRange=[3 3]  outScalingMode=Treat bit field as an integer
  Extract Bits3 : simulink/Logic and Bit Operations/Extract Bits  SystemSampleTime=-1  bitsToExtract=Range of bits  numBits=8  bitIdxRange=[2 2]  outScalingMode=Treat bit field as an integer
  Extract Bits4 : simulink/Logic and Bit Operations/Extract Bits  SystemSampleTime=-1  bitsToExtract=Range of bits  numBits=8  bitIdxRange=[1 1]  outScalingMode=Treat bit field as an integer
  Extract Bits5 : simulink/Logic and Bit Operations/Extract Bits  SystemSampleTime=-1  bitsToExtract=Range of bits  numBits=8  bitIdxRange=[0 0]  outScalingMode=Treat bit field as an integer
  Out1 : Outport
  Out2 : Outport  Port=2
  Out3 : Outport  Port=3
  Out4 : Outport  Port=4
  Out5 : Outport  Port=5
  Out6 : Outport  Port=6
  wires:
  Extract Bits5/1 -> Out1/1
  Extract Bits4/1 -> Out2/1
  Extract Bits3/1 -> Out3/1
  Extract Bits2/1 -> Out4/1
  In1/1 -> Extract Bits1/1, Extract Bits2/1, Extract Bits3/1, Extract Bits5/1, Extract Bits4/1, Extract Bits/1
  Extract Bits1/1 -> Out5/1
  Extract Bits/1 -> Out6/1

== system basis3/corr1/mux ==
  In1 : Inport
  In2 : Inport  Port=2
  C : MultiPortSwitch  Inputs=64  zeroidx=on  SampleTime=1
  Demux3 : Demux  Outputs=64
  Out1 : Outport
  wires:
  C/1 -> Out1/1
  In2/1 -> Demux3/1
  In1/1 -> C/1
  Demux3/1 -> C/2
  Demux3/2 -> C/3
  Demux3/3 -> C/4
  Demux3/4 -> C/5
  Demux3/5 -> C/6
  Demux3/6 -> C/7
  Demux3/7 -> C/8
  Demux3/8 -> C/9
  Demux3/9 -> C/10
  Demux3/10 -> C/11
  Demux3/11 -> C/12
  Demux3/12 -> C/13
  Demux3/13 -> C/14
  Demux3/15 -> C/16
  Demux3/16 -> C/17
  Demux3/17 -> C/18
  Demux3/18 -> C/19
  Demux3/19 -> C/20
  Demux3/20 -> C/21
  Demux3/21 -> C/22
  Demux3/22 -> C/23
  Demux3/23 -> C/24
  Demux3/24 -> C/25
  Demux3/25 -> C/26
  Demux3/26 -> C/27
  Demux3/27 -> C/28
  Demux3/28 -> C/29
  Demux3/29 -> C/30
  Demux3/30 -> C/31
  Demux3/31 -> C/32
  Demux3/32 -> C/33
  Demux3/33 -> C/34
  Demux3/34 -> C/35
  Demux3/35 -> C/36
  Demux3/36 -> C/37
  Demux3/37 -> C/38
  Demux3/38 -> C/39
  Demux3/39 -> C/40
  Demux3/40 -> C/41
  Demux3/41 -> C/42
  Demux3/42 -> C/43
  Demux3/43 -> C/44
  Demux3/44 -> C/45
  Demux3/45 -> C/46
  Demux3/46 -> C/47
  Demux3/47 -> C/48
  Demux3/48 -> C/49
  Demux3/49 -> C/50
  Demux3/50 -> C/51
  Demux3/51 -> C/52
  Demux3/52 -> C/53
  Demux3/53 -> C/54
  Demux3/54 -> C/55
  Demux3/55 -> C/56
  Demux3/56 -> C/57
  Demux3/57 -> C/58
  Demux3/58 -> C/59
  Demux3/59 -> C/60
  Demux3/60 -> C/61
  Demux3/61 -> C/62
  Demux3/62 -> C/63
  Demux3/63 -> C/64
  Demux3/64 -> C/65
  Demux3/14 -> C/15

== system basis3/corr2/mux ==
  In1 : Inport
  In2 : Inport  Port=2
  C : MultiPortSwitch  Inputs=64  zeroidx=on  SampleTime=1
  Demux3 : Demux  Outputs=64
  Out1 : Outport
  wires:
  C/1 -> Out1/1
  In2/1 -> Demux3/1
  In1/1 -> C/1
  Demux3/1 -> C/2
  Demux3/2 -> C/3
  Demux3/3 -> C/4
  Demux3/4 -> C/5
  Demux3/5 -> C/6
  Demux3/6 -> C/7
  Demux3/7 -> C/8
  Demux3/8 -> C/9
  Demux3/9 -> C/10
  Demux3/10 -> C/11
  Demux3/11 -> C/12
  Demux3/12 -> C/13
  Demux3/13 -> C/14
  Demux3/15 -> C/16
  Demux3/16 -> C/17
  Demux3/17 -> C/18
  Demux3/18 -> C/19
  Demux3/19 -> C/20
  Demux3/20 -> C/21
  Demux3/21 -> C/22
  Demux3/22 -> C/23
  Demux3/23 -> C/24
  Demux3/24 -> C/25
  Demux3/25 -> C/26
  Demux3/26 -> C/27
  Demux3/27 -> C/28
  Demux3/28 -> C/29
  Demux3/29 -> C/30
  Demux3/30 -> C/31
  Demux3/31 -> C/32
  Demux3/32 -> C/33
  Demux3/33 -> C/34
  Demux3/34 -> C/35
  Demux3/35 -> C/36
  Demux3/36 -> C/37
  Demux3/37 -> C/38
  Demux3/38 -> C/39
  Demux3/39 -> C/40
  Demux3/40 -> C/41
  Demux3/41 -> C/42
  Demux3/42 -> C/43
  Demux3/43 -> C/44
  Demux3/44 -> C/45
  Demux3/45 -> C/46
  Demux3/46 -> C/47
  Demux3/47 -> C/48
  Demux3/48 -> C/49
  Demux3/49 -> C/50
  Demux3/50 -> C/51
  Demux3/51 -> C/52
  Demux3/52 -> C/53
  Demux3/53 -> C/54
  Demux3/54 -> C/55
  Demux3/55 -> C/56
  Demux3/56 -> C/57
  Demux3/57 -> C/58
  Demux3/58 -> C/59
  Demux3/59 -> C/60
  Demux3/60 -> C/61
  Demux3/61 -> C/62
  Demux3/62 -> C/63
  Demux3/63 -> C/64
  Demux3/64 -> C/65
  Demux3/14 -> C/15

== system basis3/corr3/mux ==
  In1 : Inport
  In2 : Inport  Port=2
  C : MultiPortSwitch  Inputs=64  zeroidx=on  SampleTime=1
  Demux3 : Demux  Outputs=64
  Out1 : Outport
  wires:
  C/1 -> Out1/1
  In2/1 -> Demux3/1
  In1/1 -> C/1
  Demux3/1 -> C/2
  Demux3/2 -> C/3
  Demux3/3 -> C/4
  Demux3/4 -> C/5
  Demux3/5 -> C/6
  Demux3/6 -> C/7
  Demux3/7 -> C/8
  Demux3/8 -> C/9
  Demux3/9 -> C/10
  Demux3/10 -> C/11
  Demux3/11 -> C/12
  Demux3/12 -> C/13
  Demux3/13 -> C/14
  Demux3/15 -> C/16
  Demux3/16 -> C/17
  Demux3/17 -> C/18
  Demux3/18 -> C/19
  Demux3/19 -> C/20
  Demux3/20 -> C/21
  Demux3/21 -> C/22
  Demux3/22 -> C/23
  Demux3/23 -> C/24
  Demux3/24 -> C/25
  Demux3/25 -> C/26
  Demux3/26 -> C/27
  Demux3/27 -> C/28
  Demux3/28 -> C/29
  Demux3/29 -> C/30
  Demux3/30 -> C/31
  Demux3/31 -> C/32
  Demux3/32 -> C/33
  Demux3/33 -> C/34
  Demux3/34 -> C/35
  Demux3/35 -> C/36
  Demux3/36 -> C/37
  Demux3/37 -> C/38
  Demux3/38 -> C/39
  Demux3/39 -> C/40
  Demux3/40 -> C/41
  Demux3/41 -> C/42
  Demux3/42 -> C/43
  Demux3/43 -> C/44
  Demux3/44 -> C/45
  Demux3/45 -> C/46
  Demux3/46 -> C/47
  Demux3/47 -> C/48
  Demux3/48 -> C/49
  Demux3/49 -> C/50
  Demux3/50 -> C/51
  Demux3/51 -> C/52
  Demux3/52 -> C/53
  Demux3/53 -> C/54
  Demux3/54 -> C/55
  Demux3/55 -> C/56
  Demux3/56 -> C/57
  Demux3/57 -> C/58
  Demux3/58 -> C/59
  Demux3/59 -> C/60
  Demux3/60 -> C/61
  Demux3/61 -> C/62
  Demux3/62 -> C/63
  Demux3/63 -> C/64
  Demux3/64 -> C/65
  Demux3/14 -> C/15

== system basis3/pos/ws ==
  in0 : Inport
  in1 : Inport  Port=2
  in2 : Inport  Port=3
  Sum : Sum  Inputs=+++++++  SaturateOnIntegerOverflow=on  InputSameDT=on
  Out1 : Outport
  wires:
  Sum/1 -> Out1/1
  in0/1 -> Sum/1
  in1/1 -> Sum/2, Sum/3
  in2/1 -> Sum/4, Sum/5, Sum/6, Sum/7

== system basis3/basisgenerator/indgen0/ws ==
  In1 : Inport
  In2 : Inport  Port=2
  Sum : Sum  Inputs=+++  SaturateOnIntegerOverflow=on  InputSameDT=on
  Out1 : Outport
  wires:
  In1/1 -> Sum/2, Sum/1
  In2/1 -> Sum/3
  Sum/1 -> Out1/1

== system basis3/basisgenerator/indgen0/ws1 ==
  In1 : Inport
  In2 : Inport  Port=2
  Sum : Sum  Inputs=+++  SaturateOnIntegerOverflow=on  InputSameDT=on
  Out1 : Outport
  wires:
  In1/1 -> Sum/2, Sum/1
  In2/1 -> Sum/3
  Sum/1 -> Out1/1

== system basis3/basisgenerator/indgen0/ws2 ==
  In1 : Inport
  In2 : Inport  Port=2
  Sum : Sum  Inputs=+++  SaturateOnIntegerOverflow=on  InputSameDT=on
  Out1 : Outport
  wires:
  In1/1 -> Sum/2, Sum/1
  In2/1 -> Sum/3
  Sum/1 -> Out1/1

== system basis3/basisgenerator/indgen0/ws3 ==
  In1 : Inport
  In2 : Inport  Port=2
  Sum : Sum  Inputs=+++  SaturateOnIntegerOverflow=on  InputSameDT=on
  Out1 : Outport
  wires:
  In1/1 -> Sum/2, Sum/1
  In2/1 -> Sum/3
  Sum/1 -> Out1/1

== system basis3/basisgenerator/indgen1/ws ==
  In1 : Inport
  In2 : Inport  Port=2
  Sum : Sum  Inputs=+++  SaturateOnIntegerOverflow=on  InputSameDT=on
  Out1 : Outport
  wires:
  In1/1 -> Sum/2, Sum/1
  In2/1 -> Sum/3
  Sum/1 -> Out1/1

== system basis3/basisgenerator/indgen1/ws1 ==
  In1 : Inport
  In2 : Inport  Port=2
  Sum : Sum  Inputs=+++  SaturateOnIntegerOverflow=on  InputSameDT=on
  Out1 : Outport
  wires:
  In1/1 -> Sum/2, Sum/1
  In2/1 -> Sum/3
  Sum/1 -> Out1/1

== system basis3/basisgenerator/indgen1/ws2 ==
  In1 : Inport
  In2 : Inport  Port=2
  Sum : Sum  Inputs=+++  SaturateOnIntegerOverflow=on  InputSameDT=on
  Out1 : Outport
  wires:
  In1/1 -> Sum/2, Sum/1
  In2/1 -> Sum/3
  Sum/1 -> Out1/1

== system basis3/basisgenerator/indgen1/ws3 ==
  In1 : Inport
  In2 : Inport  Port=2
  Sum : Sum  Inputs=+++  SaturateOnIntegerOverflow=on  InputSameDT=on
  Out1 : Outport
  wires:
  In1/1 -> Sum/2, Sum/1
  In2/1 -> Sum/3
  Sum/1 -> Out1/1

== system basis3/basisgenerator/indgen2/ws ==
  In1 : Inport
  In2 : Inport  Port=2
  Sum : Sum  Inputs=+++  SaturateOnIntegerOverflow=on  InputSameDT=on
  Out1 : Outport
  wires:
  In1/1 -> Sum/2, Sum/1
  In2/1 -> Sum/3
  Sum/1 -> Out1/1

== system basis3/basisgenerator/indgen2/ws1 ==
  In1 : Inport
  In2 : Inport  Port=2
  Sum : Sum  Inputs=+++  SaturateOnIntegerOverflow=on  InputSameDT=on
  Out1 : Outport
  wires:
  In1/1 -> Sum/2, Sum/1
  In2/1 -> Sum/3
  Sum/1 -> Out1/1

== system basis3/basisgenerator/indgen2/ws2 ==
  In1 : Inport
  In2 : Inport  Port=2
  Sum : Sum  Inputs=+++  SaturateOnIntegerOverflow=on  InputSameDT=on
  Out1 : Outport
  wires:
  In1/1 -> Sum/2, Sum/1
  In2/1 -> Sum/3
  Sum/1 -> Out1/1

== system basis3/basisgenerator/indgen2/ws3 ==
  In1 : Inport
  In2 : Inport  Port=2
  Sum : Sum  Inputs=+++  SaturateOnIntegerOverflow=on  InputSameDT=on
  Out1 : Outport
  wires:
  In1/1 -> Sum/2, Sum/1
  In2/1 -> Sum/3
  Sum/1 -> Out1/1

== system basis3/basisgenerator1/indgen0/ws ==
  In1 : Inport
  In2 : Inport  Port=2
  Sum : Sum  Inputs=+++  SaturateOnIntegerOverflow=on  InputSameDT=on
  Out1 : Outport
  wires:
  In1/1 -> Sum/2, Sum/1
  In2/1 -> Sum/3
  Sum/1 -> Out1/1

== system basis3/basisgenerator1/indgen0/ws1 ==
  In1 : Inport
  In2 : Inport  Port=2
  Sum : Sum  Inputs=+++  SaturateOnIntegerOverflow=on  InputSameDT=on
  Out1 : Outport
  wires:
  In1/1 -> Sum/2, Sum/1
  In2/1 -> Sum/3
  Sum/1 -> Out1/1

== system basis3/basisgenerator1/indgen0/ws2 ==
  In1 : Inport
  In2 : Inport  Port=2
  Sum : Sum  Inputs=+++  SaturateOnIntegerOverflow=on  InputSameDT=on
  Out1 : Outport
  wires:
  In1/1 -> Sum/2, Sum/1
  In2/1 -> Sum/3
  Sum/1 -> Out1/1

== system basis3/basisgenerator1/indgen0/ws3 ==
  In1 : Inport
  In2 : Inport  Port=2
  Sum : Sum  Inputs=+++  SaturateOnIntegerOverflow=on  InputSameDT=on
  Out1 : Outport
  wires:
  In1/1 -> Sum/2, Sum/1
  In2/1 -> Sum/3
  Sum/1 -> Out1/1

== system basis3/basisgenerator1/indgen1/ws ==
  In1 : Inport
  In2 : Inport  Port=2
  Sum : Sum  Inputs=+++  SaturateOnIntegerOverflow=on  InputSameDT=on
  Out1 : Outport
  wires:
  In1/1 -> Sum/2, Sum/1
  In2/1 -> Sum/3
  Sum/1 -> Out1/1

== system basis3/basisgenerator1/indgen1/ws1 ==
  In1 : Inport
  In2 : Inport  Port=2
  Sum : Sum  Inputs=+++  SaturateOnIntegerOverflow=on  InputSameDT=on
  Out1 : Outport
  wires:
  In1/1 -> Sum/2, Sum/1
  In2/1 -> Sum/3
  Sum/1 -> Out1/1

== system basis3/basisgenerator1/indgen1/ws2 ==
  In1 : Inport
  In2 : Inport  Port=2
  Sum : Sum  Inputs=+++  SaturateOnIntegerOverflow=on  InputSameDT=on
  Out1 : Outport
  wires:
  In1/1 -> Sum/2, Sum/1
  In2/1 -> Sum/3
  Sum/1 -> Out1/1

== system basis3/basisgenerator1/indgen1/ws3 ==
  In1 : Inport
  In2 : Inport  Port=2
  Sum : Sum  Inputs=+++  SaturateOnIntegerOverflow=on  InputSameDT=on
  Out1 : Outport
  wires:
  In1/1 -> Sum/2, Sum/1
  In2/1 -> Sum/3
  Sum/1 -> Out1/1

== system basis3/basisgenerator1/indgen2/ws ==
  In1 : Inport
  In2 : Inport  Port=2
  Sum : Sum  Inputs=+++  SaturateOnIntegerOverflow=on  InputSameDT=on
  Out1 : Outport
  wires:
  In1/1 -> Sum/2, Sum/1
  In2/1 -> Sum/3
  Sum/1 -> Out1/1

== system basis3/basisgenerator1/indgen2/ws1 ==
  In1 : Inport
  In2 : Inport  Port=2
  Sum : Sum  Inputs=+++  SaturateOnIntegerOverflow=on  InputSameDT=on
  Out1 : Outport
  wires:
  In1/1 -> Sum/2, Sum/1
  In2/1 -> Sum/3
  Sum/1 -> Out1/1

== system basis3/basisgenerator1/indgen2/ws2 ==
  In1 : Inport
  In2 : Inport  Port=2
  Sum : Sum  Inputs=+++  SaturateOnIntegerOverflow=on  InputSameDT=on
  Out1 : Outport
  wires:
  In1/1 -> Sum/2, Sum/1
  In2/1 -> Sum/3
  Sum/1 -> Out1/1

== system basis3/basisgenerator1/indgen2/ws3 ==
  In1 : Inport
  In2 : Inport  Port=2
  Sum : Sum  Inputs=+++  SaturateOnIntegerOverflow=on  InputSameDT=on
  Out1 : Outport
  wires:
  In1/1 -> Sum/2, Sum/1
  In2/1 -> Sum/3
  Sum/1 -> Out1/1
